simulink model "main"  (R2014b)
settings: Solver=ode45  StartTime=0.0  StopTime=10.0  RelTol=1e-3
libraries: vexarmcortexlib x16
settings Model: Creator=Chase  LastModifiedBy=Chase

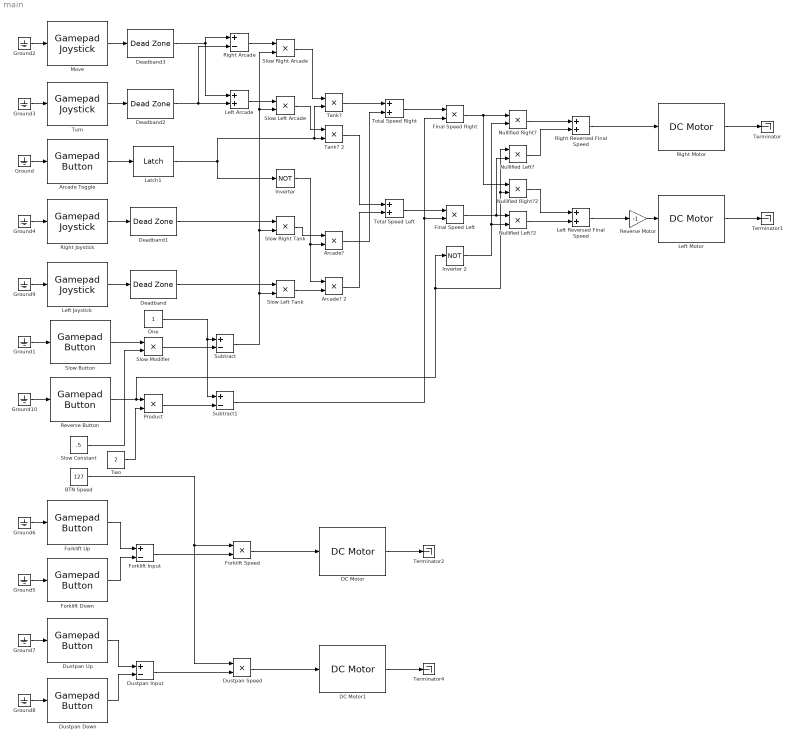
== system main ==
  Arcade Toggle : vexarmcortexlib/Gamepad Button  joystick=1  chan=5  button56=Down  button78=Right
  Arcade? : Product  RndMeth=Zero
  Arcade? 2 : Product  RndMeth=Zero
  "BTN Speed " : Constant  Value=127
  DC Motor : vexarmcortexlib/DC Motor  motor=3  scaleFactor=1/13.5
  DC Motor1 : vexarmcortexlib/DC Motor  motor=8  scaleFactor=1/13.5
  Deadband{,1..3} (4 alike) : DeadZone  LowerValue=-10  UpperValue=10  SaturateOnIntegerOverflow=on
  Dustpan Down : vexarmcortexlib/Gamepad Button  joystick=1  chan=7  button56=Down  button78=Down
  Dustpan Input : Sum  Inputs=+-
  Dustpan Speed : Product  RndMeth=Zero
  Dustpan Up : vexarmcortexlib/Gamepad Button  joystick=1  chan=7  button56=Down  button78=Up
  Final Speed Left : Product  RndMeth=Zero
  Final Speed Right : Product  RndMeth=Zero
  Forklift Down : vexarmcortexlib/Gamepad Button  joystick=1  chan=8  button56=Up  button78=Down
  Forklift Input : Sum  Inputs=+-
  Forklift Speed : Product  RndMeth=Zero
  Forklift Up : vexarmcortexlib/Gamepad Button  joystick=1  chan=8  button56=Up  button78=Up
  Ground{,1..10} (11 alike) : Ground
  Inverter : Logic  Operator=NOT  AllPortsSameDT=off  OutDataTypeStr=boolean
  "Inverter 2 " : Logic  Operator=NOT  AllPortsSameDT=off  OutDataTypeStr=boolean
  Latch1 : vexarmcortexlib/Utilities/Latch  output0=off
  Left Arcade : Sum
  Left Joystick : vexarmcortexlib/Gamepad Joystick  joystick=1  chan=3
  Left Motor : vexarmcortexlib/DC Motor  motor=1  scaleFactor=1/13.5
  Left Reversed Final Speed : Sum
  Move : vexarmcortexlib/Gamepad Joystick  joystick=1  chan=3
  Nullified Left? : Product  RndMeth=Zero
  Nullified Left?2 : Product  RndMeth=Zero
  Nullified Right? : Product  RndMeth=Zero
  Nullified Right?2 : Product  RndMeth=Zero
  One : Constant
  Product : Product
  Reverse Button : vexarmcortexlib/Gamepad Button  joystick=1  chan=6  button56=Up  button78=Right
  Reverse Motor : Gain  Gain=-1
  Right Arcade : Sum  Inputs=+-
  Right Joystick : vexarmcortexlib/Gamepad Joystick  joystick=1  chan=2
  Right Motor : vexarmcortexlib/DC Motor  motor=9  scaleFactor=1/13.5
  Right Reversed Final Speed : Sum
  Slow Button : vexarmcortexlib/Gamepad Button  joystick=1  chan=5  button56=Up  button78=Up
  Slow Constant : Constant  Value=.5
  Slow Left Arcade : Product  RndMeth=Zero
  Slow Left Tank : Product  RndMeth=Zero
  Slow Modifier : Product  RndMeth=Zero
  Slow Right Arcade : Product  RndMeth=Zero
  Slow Right Tank : Product  RndMeth=Zero
  Subtract : Sum  Inputs=+-
  Subtract1 : Sum  Inputs=+-
  Tank? : Product  RndMeth=Zero
  Tank? 2 : Product  RndMeth=Zero
  Terminator{,1..2,4} (4 alike) : Terminator
  Total Speed Left : Sum
  Total Speed Right : Sum
  Turn : vexarmcortexlib/Gamepad Joystick  joystick=1  chan=1
  Two : Constant  Value=2
  wires:
  Right Motor/1 -> Terminator/1
  Left Motor/1 -> Terminator1/1
  Left Joystick/1 -> Deadband/1
  Right Joystick/1 -> Deadband1/1
  Ground5/1 -> Forklift Down/1
  Ground6/1 -> Forklift Up/1
  Forklift Up/1 -> Forklift Input/1
  Forklift Down/1 -> Forklift Input/2
  Ground7/1 -> Dustpan Up/1
  Ground8/1 -> Dustpan Down/1
  Dustpan Up/1 -> Dustpan Input/1
  Dustpan Down/1 -> Dustpan Input/2
  Latch1/1 -> Inverter/1, Tank?/2, Tank? 2/2
  Arcade Toggle/1 -> Latch1/1
  Ground/1 -> Arcade Toggle/1
  Move/1 -> Deadband3/1
  Turn/1 -> Deadband2/1
  Deadband3/1 -> Right Arcade/1, Left Arcade/1
  Deadband2/1 -> Left Arcade/2, Right Arcade/2
  "BTN Speed "/1 -> Dustpan Speed/1, Forklift Speed/1
  Forklift Input/1 -> Forklift Speed/2
  Dustpan Input/1 -> Dustpan Speed/2
  Dustpan Speed/1 -> DC Motor1/1
  Forklift Speed/1 -> DC Motor/1
  DC Motor/1 -> Terminator2/1
  DC Motor1/1 -> Terminator4/1
  Ground1/1 -> Slow Button/1
  Slow Button/1 -> Slow Modifier/1
  Slow Constant/1 -> Slow Modifier/2
  Left Arcade/1 -> Slow Left Arcade/1
  Right Arcade/1 -> Slow Right Arcade/1
  Deadband1/1 -> Slow Right Tank/1
  Deadband/1 -> Slow Left Tank/1
  Ground2/1 -> Move/1
  Ground3/1 -> Turn/1
  Ground4/1 -> Right Joystick/1
  Ground9/1 -> Left Joystick/1
  Reverse Motor/1 -> Left Motor/1
  Slow Left Tank/1 -> Arcade? 2/2
  Slow Left Arcade/1 -> Tank? 2/1
  Slow Right Arcade/1 -> Tank?/1
  Inverter/1 -> Arcade?/2, Arcade? 2/1
  Slow Right Tank/1 -> Arcade?/1
  Arcade?/1 -> Total Speed Right/2
  Arcade? 2/1 -> Total Speed Left/2
  Tank? 2/1 -> Total Speed Left/1
  Tank?/1 -> Total Speed Right/1
  Ground10/1 -> Reverse Button/1
  Total Speed Left/1 -> Final Speed Left/1
  Total Speed Right/1 -> Final Speed Right/1
  Slow Modifier/1 -> Subtract/2
  One/1 -> Subtract1/1, Subtract/1
  Subtract/1 -> Slow Right Tank/2, Slow Right Arcade/2, Slow Left Arcade/2, Slow Left Tank/2
  Reverse Button/1 -> "Inverter 2 "/1, Nullified Right?2/2, Nullified Left?/1, Product/1
  Two/1 -> Product/2
  Product/1 -> Subtract1/2
  Subtract1/1 -> Final Speed Right/2, Final Speed Left/2
  "Inverter 2 "/1 -> Nullified Right?/2, Nullified Left?2/2
  Final Speed Left/1 -> Nullified Left?2/1, Nullified Left?/2
  Final Speed Right/1 -> Nullified Right?2/1, Nullified Right?/1
  Right Reversed Final Speed/1 -> Right Motor/1
  Nullified Right?/1 -> Right Reversed Final Speed/1
  Nullified Left?/1 -> Right Reversed Final Speed/2
  Nullified Right?2/1 -> Left Reversed Final Speed/1
  Nullified Left?2/1 -> Left Reversed Final Speed/2
  Left Reversed Final Speed/1 -> Reverse Motor/1
